simulink model "deadReckon"  (R2023a)
settings: Solver=FixedStepDiscrete  StartTime=0.0  StopTime=10  FixedStep=0.01  RelTol=1e-3
model workspace (MAT data in the model file):
  ticksPerRot = 360
  wheelR = 0.052
libraries: mobileRoboticsTrainingLib x3
settings Model: Creator=khydf  LastModifiedBy=khydf

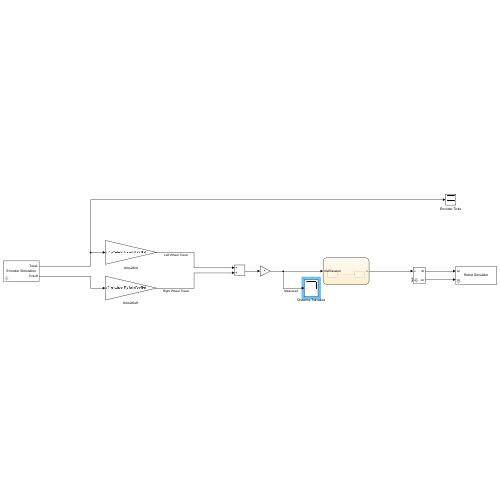
[thumbnail: Simulink's stored preview of the top-level diagram]
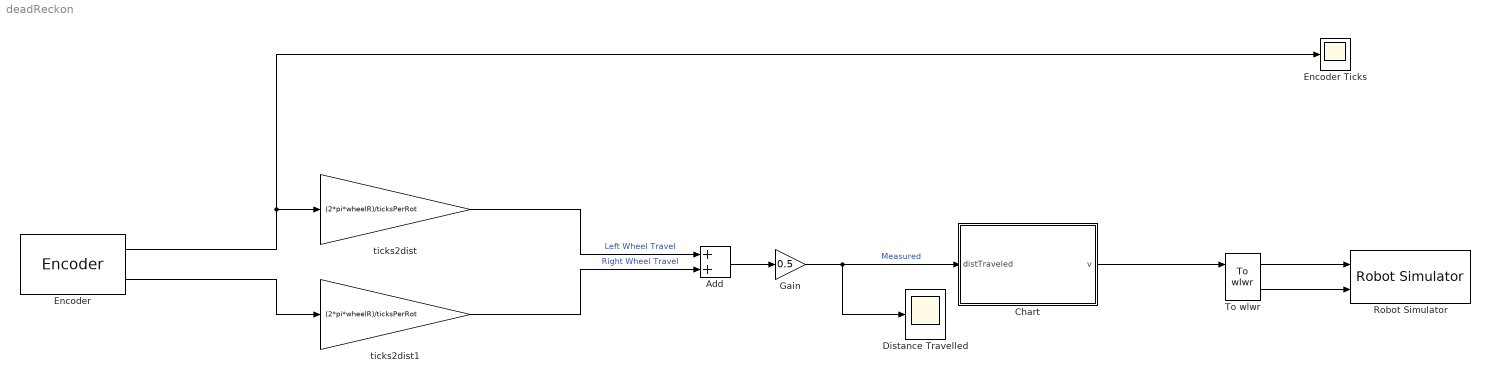
== system deadReckon ==
  Add : Sum
  Chart : Stateflow chart  TreatAsAtomicUnit=on
  Distance Travelled : Scope
  Encoder : mobileRoboticsTrainingLib/Encoder  axleLength=axleLength  wheelR=wheelR  ticksPerRot=ticksPerRot
      settings: SourceProductName=Mobile Robotics Training Library
  Encoder Ticks : Scope
  Gain : Gain  Gain=0.5
  Robot Simulator : mobileRoboticsTrainingLib/Robot Simulator  Priority=99  mapVar=[]  startX=0  startY=1  startTheta=0  axleLength=axleLength  wheelR=wheelR
  To wlwr : mobileRoboticsTrainingLib/To wlwr  axleLength=axleLength  wheelR=wheelR
  ticks2dist : Gain  Gain=(2*pi*wheelR)/ticksPerRot
  ticks2dist1 : Gain  Gain=(2*pi*wheelR)/ticksPerRot
  wires:
  Encoder/1 -> ticks2dist/1, Encoder Ticks/1
  ticks2dist/1 -> Add/1  "Left Wheel Travel"
  ticks2dist1/1 -> Add/2  "Right Wheel Travel"
  Encoder/2 -> ticks2dist1/1
  Add/1 -> Gain/1
  Gain/1 -> Distance Travelled/1, Chart/1(distTraveled)  "Measured"
  Chart/1(v) -> To wlwr/1
  To wlwr/1 -> Robot Simulator/1
  To wlwr/2 -> Robot Simulator/2

== stateflow chart deadReckon/Chart ==
  state MoveForward
    v = 0.1
  state Stop
    v = 0
  (default) -> MoveForward : %Start
  MoveForward -> Stop : [distTraveled >= 1]
  data: distTraveled input; v output
